simulink model "DigitizingDesign"  (R2014b)
settings: Solver=FixedStepDiscrete  StartTime=0.0  StopTime=2050  FixedStep=1  RelTol=1e-3
InitFcn:
  | initialize;
StopFcn:
  | stopscript
libraries: BlockLib x13, dspsrcs4 x1
settings Model: Creator=kunalmenda  LastModifiedBy=kunalmenda
settings SolverCC: AlgebraicLoopSolver=LineSearch

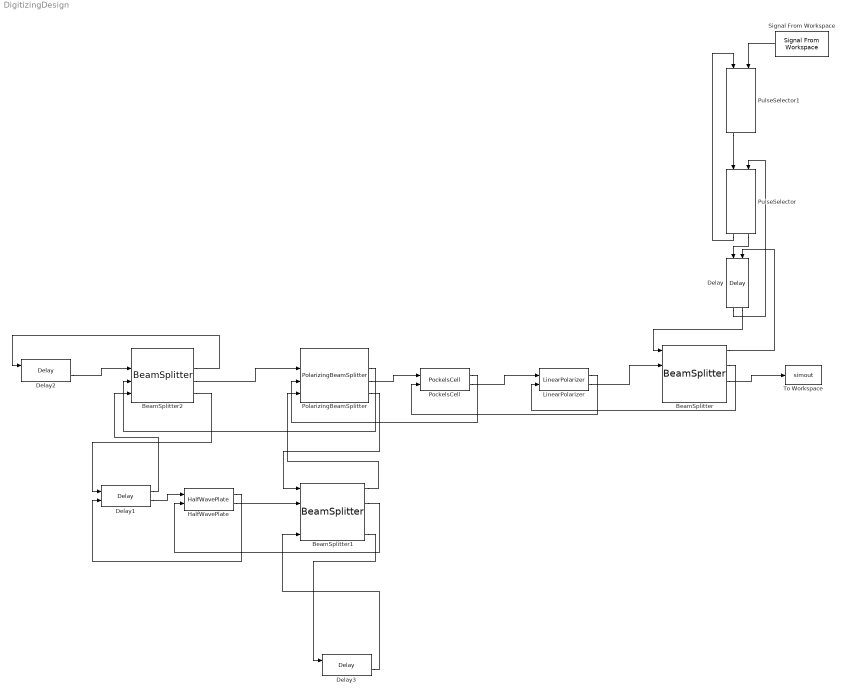
== system DigitizingDesign ==
  BeamSplitter : BlockLib/BeamSplitter  Transmittance=0.50  Reflectance=0.50  Ghost=0  BackReflectance=0.001
  BeamSplitter1 : BlockLib/BeamSplitter  Transmittance=0.50  Reflectance=0.50  Ghost=0.005  BackReflectance=0.001
  BeamSplitter2 : BlockLib/BeamSplitter  Transmittance=0.50  Reflectance=0.50  Ghost=0.005  BackReflectance=0.001
  Delay : BlockLib/Delay  DelayAmt=0
  Delay1 : BlockLib/Delay  DelayAmt=1.3227e-08
  Delay2 : BlockLib/Delay  DelayAmt=1.3000e-08
  Delay3 : BlockLib/Delay  DelayAmt=1.9664e-08
  HalfWavePlate : BlockLib/HalfWavePlate  Psi=pi/4  Transmittence=1
  LinearPolarizer : BlockLib/LinearPolarizer  Psi=pi/2  Transmittence=0.81  ExtinctionRatio=200000000
  PockelsCell : BlockLib/PockelsCell  PCTimings="[0.0103    0.1236    0.1647    0.2006]*1e-5"  ControlPowers=[1,1]  Psi=pi/4
  PolarizingBeamSplitter : BlockLib/PolarizingBeamSplitter  Psi=pi/2  Transmittance=0.50  Reflectance=0.50  Ghost=0.005  BackReflectance=0.001
  PulseSelector : BlockLib/PulseSelector  PCTimings="[0.0012    0.0014    0.0103    0.0105    0.0376    0.0378    0.0779    0.0781    0.1234    0.1236  0.1637    0.1639    0.1910    0.1912    0.2014    0.2016]*1e-5"  ControlPowers="[0.5000,    1.0000,    1.0000,    1.0000, 1.0000,    1.0000,    1.0000,    0.5000]"
  PulseSelector1 : BlockLib/PulseSelector  PCTimings="[0.0012    0.0014    0.0103    0.0105    0.0376    0.0378    0.0779    0.0781    0.1234    0.1236  0.1637    0.1639    0.1910    0.1912    0.2014    0.2016]*1e-5"  ControlPowers="[0.5000    1.0000    1.0000    1.0000    1.0000    1.0000    1.0000    0.5000]"
  Signal From Workspace : dspsrcs4/Signal From Workspace  X=inputsignal  Ts=1  nsamps=1  OutputAfterFinalValue=Setting to zero  ignoreOrWarnInputAndFrameLengths=off
  To Workspace : ToWorkspace  VariableName=simout  SaveFormat=Timeseries  SampleTime=-1
  wires:
  BeamSplitter/2 -> LinearPolarizer/2
  LinearPolarizer/1 -> PockelsCell/2
  PockelsCell/1 -> PolarizingBeamSplitter/3
  PulseSelector/2 -> Delay/1
  Delay/2 -> BeamSplitter/1
  PolarizingBeamSplitter/4 -> BeamSplitter1/1
  PolarizingBeamSplitter/2 -> BeamSplitter2/3
  BeamSplitter2/4 -> Delay1/1
  Delay1/2 -> HalfWavePlate/1
  HalfWavePlate/2 -> BeamSplitter1/2
  BeamSplitter1/2 -> HalfWavePlate/2
  HalfWavePlate/1 -> Delay1/2
  Delay1/1 -> BeamSplitter2/4
  BeamSplitter1/1 -> PolarizingBeamSplitter/4
  Delay2/2 -> BeamSplitter2/2
  BeamSplitter2/2 -> Delay2/1
  BeamSplitter2/3 -> PolarizingBeamSplitter/2
  PolarizingBeamSplitter/3 -> PockelsCell/1
  PockelsCell/2 -> LinearPolarizer/1
  LinearPolarizer/2 -> BeamSplitter/2
  BeamSplitter/3 -> To Workspace/1
  BeamSplitter1/4 -> Delay3/1
  Delay3/2 -> BeamSplitter1/4
  Delay/1 -> PulseSelector/2
  BeamSplitter/1 -> Delay/2
  Signal From Workspace/1 -> PulseSelector1/2
  PulseSelector/1 -> PulseSelector1/1
  PulseSelector1/1 -> PulseSelector/1
